simulink model "Voter_TPP"  (R2024b)
settings: Solver=VariableStepAuto  StartTime=0.0  StopTime=6  RelTol=1e-3
libraries: simulink x3
settings Model: Creator=Michele  LastModifiedBy=feder
settings ConfigComp: CovMetricSettings=dcmwe

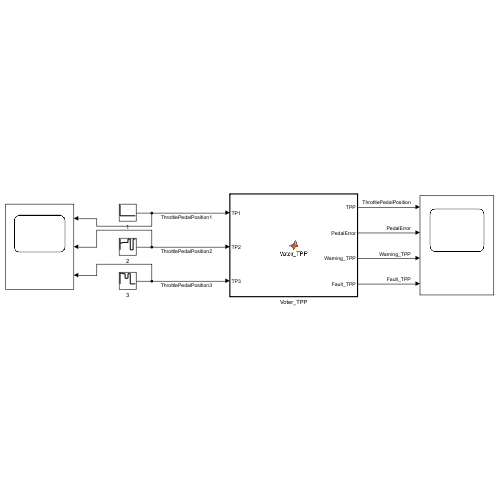
[thumbnail: Simulink's stored preview of the top-level diagram]
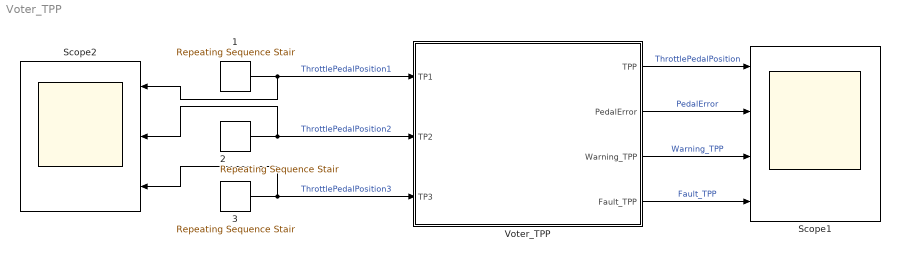
== system Voter_TPP ==
  1 : simulink/Sources/Repeating Sequence Stair  OutValues=[0.8].'  tsamp=6  OutMin=[]  OutMax=[]  OutDataTypeStr=single  OutputDataTypeScalingMode=single  OutDataType=Enum: TransmissionState  ConRadixGroup=Best Precision: Vector-wise  OutScaling=[]
  2 : simulink/Sources/Repeating Sequence Stair  OutValues=[0.8 0.81 0.81 0.9 0.62 0.9 ].'  tsamp=1  OutMin=[]  OutMax=[]  OutDataTypeStr=single  OutputDataTypeScalingMode=single  OutDataType=Enum: TransmissionState  ConRadixGroup=Best Precision: Vector-wise  OutScaling=[]
  3 : simulink/Sources/Repeating Sequence Stair  OutValues=[0.8 0.79 0.7 0.79 0.6 0.6].'  tsamp=1  OutMin=[]  OutMax=[]  OutDataTypeStr=single  OutputDataTypeScalingMode=single  OutDataType=Enum: TransmissionState  ConRadixGroup=Best Precision: Vector-wise  OutScaling=[]
  Scope1 : Scope  NumInputPorts=4
  Scope2 : Scope  NumInputPorts=3
  Voter_TPP : MATLAB Function  TreatAsAtomicUnit=on
  wires:
  3/1 -> Scope2/3, Voter_TPP/3(TP3)  "ThrottlePedalPosition3"
  Voter_TPP/1(TPP) -> Scope1/1  "ThrottlePedalPosition"
  Voter_TPP/4(Fault_TPP) -> Scope1/4  "Fault_TPP"
  Voter_TPP/3(Warning_TPP) -> Scope1/3  "Warning_TPP"
  2/1 -> Scope2/2, Voter_TPP/2(TP2)  "ThrottlePedalPosition2"
  1/1 -> Scope2/1, Voter_TPP/1(TP1)  "ThrottlePedalPosition1"
  Voter_TPP/2(PedalError) -> Scope1/2  "PedalError"

== matlab function Voter_TPP/Voter_TPP ==
  data: TPP output; PedalError output; TP1 input; Warning_TPP output Enum: WarningType; TP2 input; TP3 input; Fault_TPP output
function [TPP,PedalError,Warning_TPP,Fault_TPP] = Voter_TPP(TP1,TP2,TP3)

% Initialization of the output
TPP = single(0);
Warning_TPP = WarningType(0);
PedalError = single(0);
Fault_TPP = boolean(0);
comp = 0.02;

% Comparison between the signals
Diff_1_2 = abs(TP1-TP2);
Diff_1_3 = abs(TP1-TP3);
Diff_2_3 = abs(TP2-TP3);

if (Diff_1_2 <= comp && Diff_1_3 <= comp)

    TPP = (TP1 + TP2 + TP3)/3;
    
elseif Diff_1_2 <= comp

    TPP = (TP1 + TP2)/2;
    Warning_TPP = WarningType(1);
    PedalError = single(3);

elseif Diff_1_3 <= comp

    TPP = (TP1 + TP3)/2;
    Warning_TPP = WarningType(1);
    PedalError = single(2);

elseif Diff_2_3 <= comp

    TPP = (TP2 + TP3)/2;
    Warning_TPP = WarningType(1);
    PedalError = single(1);

else
    
    TPP = single(0);
    Warning_TPP = WarningType(2);
    Fault_TPP = boolean(1);    
    PedalError = single(4);

end
